simulink model "yoshi_rover_openloop"  (R2013b)
settings: Solver=ode3  SolverMode=SingleTasking  StartTime=0.0  StopTime=inf  RelTol=1e-3
model workspace (MAT data in the model file):
  rc = 0
  blc = -50
  brc = -50
  flc = 50
  frc = 20
undefined symbols (not defined in the file): DiscIntNeverNeededParam, sigbuilder_block, StatusID
libraries: arduinolib x5, simulink x5
settings Model: ExtModeTrigDuration=2  Creator=sbiagion  LastModifiedBy=scastro
settings DataIOCC: SignalLoggingSaveFormat=ModelDataLogs
settings OptimizationCC: OptimizeModelRefInitCode=on  LifeSpan=1
settings DebuggingCC: SolverPrmCheckMsg=none  MultiTaskDSMMsg=warning  MultiTaskCondExecSysMsg=none  StateNameClashWarn=warning
settings HardwareCC: ProdBitPerInt=16  ProdBitPerPointer=8  ProdIntDivRoundTo=Zero  ProdEndianess=LittleEndian  ProdWordSize=8  ProdHWDeviceType=Atmel->AVR
settings RTWCC: SystemTargetFile=realtime.tlc  GenerateMakefile=off  TemplateMakefile=realtime.tmf  Description=Run on Target Hardware  RTWVerbose=off  ProcessScript=realtime_make_rtw_hook  IncludeERTFirstTime=on
settings STFCustomTargetCC: TargetLibSuffix=.a  GenerateSampleERTMain=on  ERTCustomFileBanners=on  SupportNonInlinedSFcns=off  SupportVariableSizeSignals=on  MATLABClassNameForMDSCustomization=Simulink.SoftwareTarget.ERTCustomization  GRTInterface=off  SystemTargetFile=realtime.tlc
settings ERTTargetCC: CodeReplacementLibrary=ANSI_C  GenerateSampleERTMain=on  ParMdlRefBuildCompliant=off  CompOptLevelCompliant=off  ConcurrentExecutionCompliant=off  CombineOutputUpdateFcns=off  ERTFirstTimeCompliant=off  SupportContinuousTime=on  SupportVariableSizeSignals=on  ModelStepFunctionPrototypeControlCompliant=off  CPPClassGenCompliant=off  ExtModeTransport=3  ExtModeMexFile=ext_serial_win32_comm  ExtModeMexArgs=0 6 115200  InlinedParameterPlacement=NonHierarchical  ERTSrcFileBannerTemplate=realtime_code_template.cgt  ERTHdrFileBannerTemplate=realtime_code_template.cgt  ERTDataSrcFileTemplate=realtime_code_template.cgt  ERTDataHdrFileTemplate=realtime_code_template.cgt  ERTCustomFileTemplate=realtime_file_process.tlc

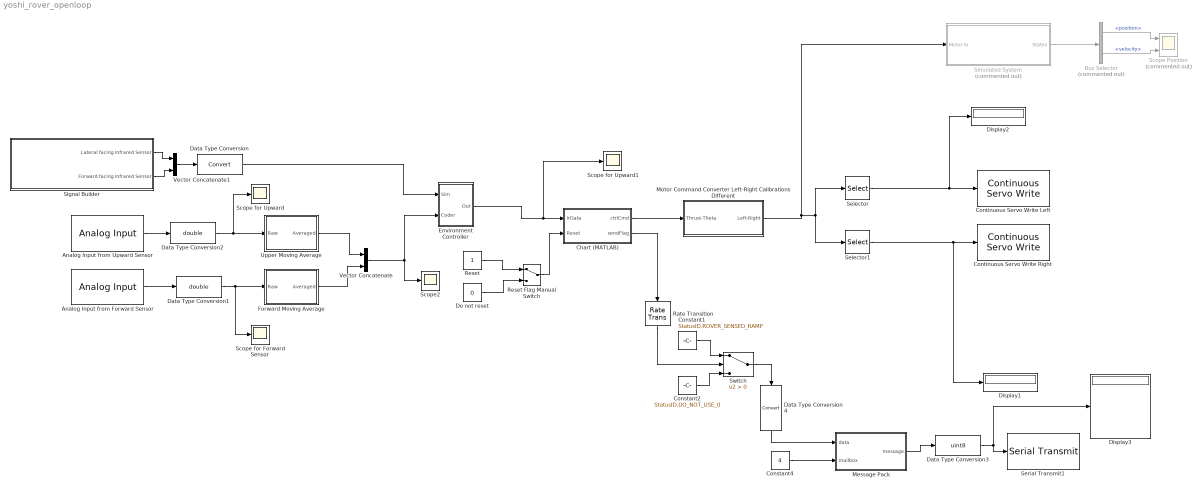
== system yoshi_rover_openloop ==
  Analog Input from Forward Sensor : arduinolib/Analog Input  pinNumber=1  sampleTime=0.01
  Analog Input from Upward Sensor : arduinolib/Analog Input  pinNumber=0  sampleTime=0.01
  Bus Selector : BusSelector  Commented=on  OutputSignals=position,velocity
  Chart (MATLAB) : Stateflow chart  TreatAsAtomicUnit=on
  Constant1 : Constant  Value=StatusID.ROVER_SENSED_RAMP  SampleTime=0.1
  Constant2 : Constant  Value=StatusID.DO_NOT_USE_0  SampleTime=0.1
  Constant4 : Constant  Value=4
  Continuous Servo Write Left : arduinolib/Continuous Servo Write  pinNumber=48
  Continuous Servo Write Right : arduinolib/Continuous Servo Write  pinNumber=49
  Data Type Conversion : DataTypeConversion
  Data Type Conversion1 : DataTypeConversion  OutDataTypeStr=double
  Data Type Conversion2 : DataTypeConversion  OutDataTypeStr=double
  Data Type Conversion3 : DataTypeConversion  OutDataTypeStr=uint8
  Data Type Conversion4 : DataTypeConversion
  Display1 : Display
  Display2 : Display
  Display3 : Display
  Do not reset : Constant  Value=0
  Environment Controller : Subsystem  mask(Environment Controller){}
      mask help: Simulink:masks:EnvironmentController_MD
      mask init:
      | switch_mode = rtwenvironmentmode(bdroot(gcbh)) || ...
      |     (exist('sldvisactive','file')~=0 && sldvisactive(bdroot(gcbh)));
  Forward Moving Average : Subsystem
  Message Pack : Subsystem
  Motor Command Converter Left-Right Calibrations Different : Subsystem  AncestorBlock="battlebots_library/Motor Control/Motor Command Converter  Left-Right Calibrations Different"  mask{fcl=flc, fcr=frc, rc=rc, bcl=blc, bcr=brc}
      mask prompts: fcl "Forward Left"; fcr "Forward Right"; rc "Rest"; bcl "Backward Left"; bcr "Backward Right"
  Rate Transition : RateTransition  OutPortSampleTime=0.1
  Reset : Constant
  Reset Flag Manual Switch : ManualSwitch
  Scope Position : Scope  Commented=on  NumInputPorts=2
      settings: ShowLegends=on  YMin=-5~-0.5  YMax=5~1  SaveName=ScopeData3
  Scope for Forward Sensor : Scope
      settings: YMin=0  YMax=1000
  Scope for Upward : Scope
      settings: YMin=25  YMax=525  SaveName=ScopeData6
  Scope for Upward1 : Scope
      settings: ShowLegends=on  YMin=0  YMax=700  SaveName=RoverSensorData
  Scope2 : Scope
      settings: ShowLegends=on  YMin=25  YMax=600  SaveName=ScopeData2
  Selector : Selector  InputPortWidth=2  IndexOptions=Index vector (dialog)  Indices=1  OutputSizes=1
  Selector1 : Selector  InputPortWidth=2  IndexOptions=Index vector (dialog)  Indices=2  OutputSizes=1
  Serial Transmit1 : arduinolib/Serial Transmit  portNumber=1
  Signal Builder : Subsystem  Tag=STV Subsys  LoadFcn=sigbuilder_block('load');  StartFcn=sigbuilder_block('start');  StopFcn=sigbuilder_block('stop');  ClipboardFcn=sigbuilder_block('clipboard');  mask(Sigbuilder block){}
      mask help: Simulink:masks:SigbuilderBlock_MD
      mask init:
      | if ~strcmp(get_param(bdroot(gcbh),'SimulationStatus'),'stopped') tuvar = sigbuilder_block('maskInit'); end
      settings: CopyFcn=sigbuilder_block('copy');  DeleteFcn=sigbuilder_block('delete');  ModelCloseFcn=sigbuilder_block('modelClose');  PreSaveFcn=sigbuilder_block('preSave');  PauseFcn=sigbuilder_block('pause');  ContinueFcn=sigbuilder_block('continue');  NameChangeFcn=sigbuilder_block('namechange');  OpenFcn=sigbuilder_block('open',[36 193.034 550.552 399.724 ]);  CloseFcn=sigbuilder_block('close');
      mask Display: plot(0, 0, 100, 100,[2, 2, 32, 32, 2], [68, 8, 8, 68, 68],[32, 2], [38, 38], [32, 19, 2],[53, 60, 44], [32, 17, 17, 2],[16, 16, 31, 31]);txt = getActiveGroup(gcbh);text(2, 100, txt,'verticalAlignment', 'top');
  Simulated System : Subsystem  Commented=on  AncestorBlock=battlebots_library/Simulation/Simulated System1  mask{max2vel=1, xm_initial_ft=0, ym_initial_ft=0, om_initial_rad=0, wheelbase_ft=1}
      mask prompts: max2vel "Gain to convert maximum command to velocity"; xm_initial_ft "Initial x position in ft"; ym_initial_ft "Initial y position in ft"; om_initial_rad "Initial orientation in radians"; wheelbase_ft "Wheelbase in ft"
  Switch : Switch  Criteria=u2 > Threshold
  Upper Moving Average : Subsystem
  Vector Concatenate : Concatenate
  Vector Concatenate1 : Concatenate
  wires:
  Analog Input from Upward Sensor/1 -> Data Type Conversion2/1
  Environment Controller/1(Out) -> Scope for Upward1/1, Chart (MATLAB)/1(irData)
  Data Type Conversion/1 -> Environment Controller/1(Sim)
  Signal Builder/2(Forward facing Infrared Sensor) -> Vector Concatenate1/2
  Signal Builder/1(Lateral facing Infrared Sensor) -> Vector Concatenate1/1
  Vector Concatenate1/1 -> Data Type Conversion/1
  Motor Command Converter Left-Right Calibrations Different/1(Left-Right) -> Simulated System/1(Motor In), Selector1/1, Selector/1
  Vector Concatenate/1 -> Scope2/1, Environment Controller/2(Coder)
  Analog Input from Forward Sensor/1 -> Data Type Conversion1/1
  Data Type Conversion2/1 -> Scope for Upward/1, Upper Moving Average/1(Raw)
  Selector1/1 -> Display1/1, Continuous Servo Write Right/1
  Selector/1 -> Continuous Servo Write Left/1, Display2/1
  Simulated System/1(States) -> Bus Selector/1
  Bus Selector/1 -> Scope Position/1  "<position>"
  Bus Selector/2 -> Scope Position/2  "<velocity>"
  Chart (MATLAB)/1(ctrlCmd) -> Motor Command Converter Left-Right Calibrations Different/1(Thrust-Theta)
  Data Type Conversion1/1 -> Scope for Forward Sensor/1, Forward Moving Average/1(Raw)
  Forward Moving Average/1("Averaged ") -> Vector Concatenate/2
  Upper Moving Average/1(Averaged) -> Vector Concatenate/1
  Reset Flag Manual Switch/1 -> Chart (MATLAB)/2(Reset)
  Reset/1 -> Reset Flag Manual Switch/1
  Do not reset/1 -> Reset Flag Manual Switch/2
  Constant4/1 -> Message Pack/2(mailbox)
  Message Pack/1(message) -> Data Type Conversion3/1
  Data Type Conversion3/1 -> Serial Transmit1/1, Display3/1
  Chart (MATLAB)/2(sendFlag) -> Rate Transition/1
  Constant1/1 -> Switch/1
  Constant2/1 -> Switch/3
  Switch/1 -> Data Type Conversion4/1
  Data Type Conversion4/1 -> Message Pack/1(data)
  Rate Transition/1 -> Switch/2

== system yoshi_rover_openloop/Environment Controller ==
  Sim : Inport
  Coder : Inport  Port=2
  Environment Switch : Switch  DisableCoverage=on  Criteria=u2 ~= 0  ZeroCross=off  InputSameDT=on
  Numerical Unity : SignalConversion
  Switch Control : Constant  DisableCoverage=on  Value=switch_mode  OutDataTypeStr=boolean
  Out : Outport
  wires:
  Numerical Unity/1 -> Out/1
  Coder/1 -> Environment Switch/3
  Environment Switch/1 -> Numerical Unity/1
  Switch Control/1 -> Environment Switch/2
  Sim/1 -> Environment Switch/1

== system yoshi_rover_openloop/Forward Moving Average ==
  Raw : Inport
  Gain : Gain  Gain=1/15
  Sum of Elements : Sum  Inputs=+
  Tapped Delay : simulink/Discrete/Tapped Delay  vinit=0.0  samptime=-1  NumDelays=15  DelayOrder=Oldest  includeCurrent=off
  "Averaged " : Outport
  wires:
  Sum of Elements/1 -> Gain/1
  Tapped Delay/1 -> Sum of Elements/1
  Gain/1 -> "Averaged "/1
  Raw/1 -> Tapped Delay/1

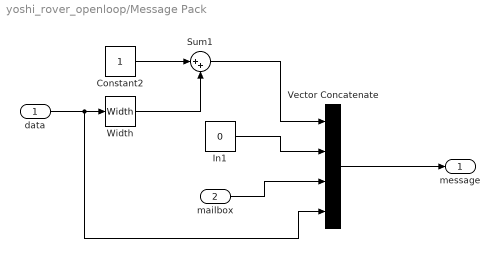
== system yoshi_rover_openloop/Message Pack ==
  data : Inport
  mailbox : Inport  Port=2
  Constant2 : Constant
  In1 : Constant  Value=0
  Sum1 : Sum  Inputs=|++
  Vector Concatenate : Concatenate  NumInputs=4
  Width : Width
  message : Outport
  wires:
  Constant2/1 -> Sum1/1
  In1/1 -> Vector Concatenate/2
  data/1 -> Vector Concatenate/4, Width/1
  Vector Concatenate/1 -> message/1
  mailbox/1 -> Vector Concatenate/3
  Sum1/1 -> Vector Concatenate/1
  Width/1 -> Sum1/2

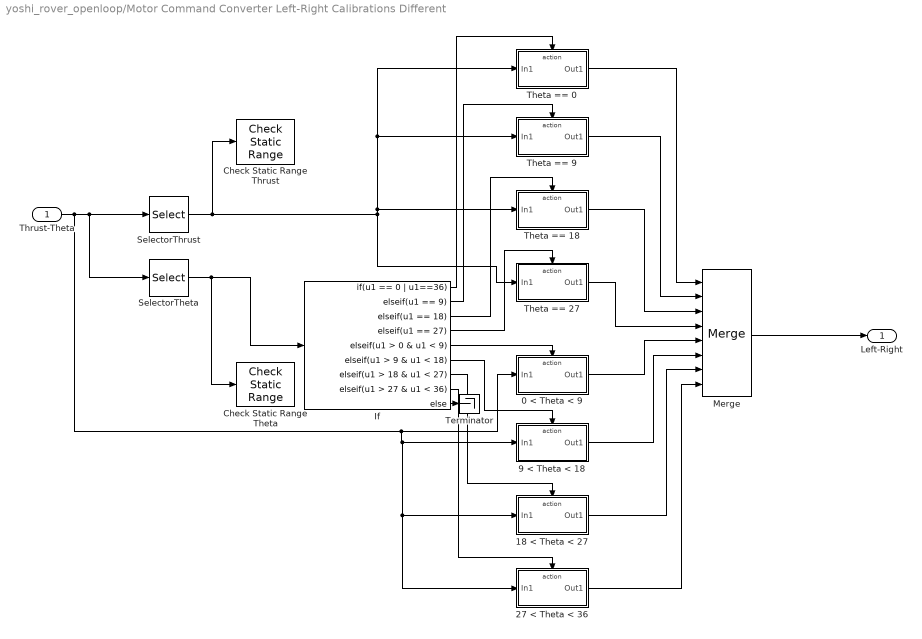
== system yoshi_rover_openloop/Motor Command Converter Left-Right Calibrations Different ==
  Thrust-Theta : Inport
  0 < Theta < 9 : Subsystem  TreatAsAtomicUnit=on
  18 < Theta < 27 : Subsystem  TreatAsAtomicUnit=on
  27 < Theta < 36 : Subsystem  TreatAsAtomicUnit=on
  9 < Theta < 18 : Subsystem  TreatAsAtomicUnit=on
  Check Static Range Theta : simulink/Model Verification/Check  Static Range  Description=0 <= u <= 36  max=36  max_included=on  min=0  min_included=on  enabled=on  callback=error('Theta Out of Range. Must be between 0 and 36, inclusively.')  stopWhenAssertionFail=on  export=off  icon=graphic
  Check Static Range Thrust : simulink/Model Verification/Check  Static Range  Description=0 <= u <= 9  max=9  max_included=on  min=0  min_included=on  enabled=on  callback=error('Thrust Out of Range. Must be between 0 and 9, inclusively.')  stopWhenAssertionFail=on  export=off  icon=graphic
  If : If  IfExpression=u1 == 0 | u1==36  ElseIfExpressions=u1 == 9, u1 == 18, u1 == 27, u1 > 0 & u1 < 9, u1 > 9 & u1 < 18, u1 > 18 & u1 < 27, u1 > 27 & u1 < 36
  Merge : Merge  Inputs=8
  "SelectorTheta " : Selector  InputPortWidth=2  IndexOptions=Index vector (dialog)  Indices=[2]  OutputSizes=1
  SelectorThrust : Selector  InputPortWidth=2  IndexOptions=Index vector (dialog)  Indices=[1]  OutputSizes=1
  Terminator : Terminator
  Theta == 0 : Subsystem  TreatAsAtomicUnit=on
  Theta == 18 : Subsystem  TreatAsAtomicUnit=on
  Theta == 27 : Subsystem  TreatAsAtomicUnit=on
  Theta == 9 : Subsystem  TreatAsAtomicUnit=on
  Left-Right : Outport
  wires:
  If/9 -> Terminator/1
  Thrust-Theta/1 -> 27 < Theta < 36/1(In1), 18 < Theta < 27/1(In1), 9 < Theta < 18/1(In1), 0 < Theta < 9/1(In1), "SelectorTheta "/1, SelectorThrust/1
  "SelectorTheta "/1 -> If/1, Check Static Range Theta/1
  If/1 -> Theta == 0/Action
  If/2 -> Theta == 9/Action
  If/3 -> Theta == 18/Action
  If/4 -> Theta == 27/Action
  If/5 -> 0 < Theta < 9/Action
  If/6 -> 9 < Theta < 18/Action
  If/7 -> 18 < Theta < 27/Action
  If/8 -> 27 < Theta < 36/Action
  SelectorThrust/1 -> Theta == 0/1(In1), Theta == 9/1(In1), Theta == 18/1(In1), Theta == 27/1(In1), Check Static Range Thrust/1
  Theta == 0/1(Out1) -> Merge/1
  Theta == 9/1(Out1) -> Merge/2
  Theta == 18/1(Out1) -> Merge/3
  Merge/1 -> Left-Right/1
  Theta == 27/1(Out1) -> Merge/4
  0 < Theta < 9/1(Out1) -> Merge/5
  9 < Theta < 18/1(Out1) -> Merge/6
  18 < Theta < 27/1(Out1) -> Merge/7
  27 < Theta < 36/1(Out1) -> Merge/8

== system yoshi_rover_openloop/Signal Builder ==
  Demux : Demux  Tag=STV Demux  Outputs=2
  FromWs : FromWorkspace  Tag=STV FromWs  VariableName=tuvar  OutputAfterFinalValue=Holding final value
      SigBuilderData=|
      | common.afterFinalStr = 'Hold final value'
      | common.sampleTime = '-1'
      | dataSet.timeRange = [0 20]
      | dataSet.name = 'Group 1'
      | sbobj.Groups.Name = 'Group 1'
      | sbobj.Groups.Signals(1).Name = 'Lateral facing Infrared Sensor'
      | sbobj.Groups.Signals(1).XData = [0 5 5 7 7 20]
      | sbobj.Groups.Signals(1).YData = [200 199.5 402 400 200 200]
      | sbobj.Groups.Signals(2).Name = 'Forward facing Infrared Sensor'
      | sbobj.Groups.Signals(2).XData = [0 12 16 20]
      | sbobj.Groups.Signals(2).YData = [200 200 450 496]
      | sbobj.Groups.TimeRange = [0 20]
  Lateral facing Infrared Sensor : Outport  Tag=STV Outport
  Forward facing Infrared Sensor : Outport  Tag=STV Outport  Port=2
  wires:
  Demux/1 -> Lateral facing Infrared Sensor/1
  FromWs/1 -> Demux/1
  Demux/2 -> Forward facing Infrared Sensor/1

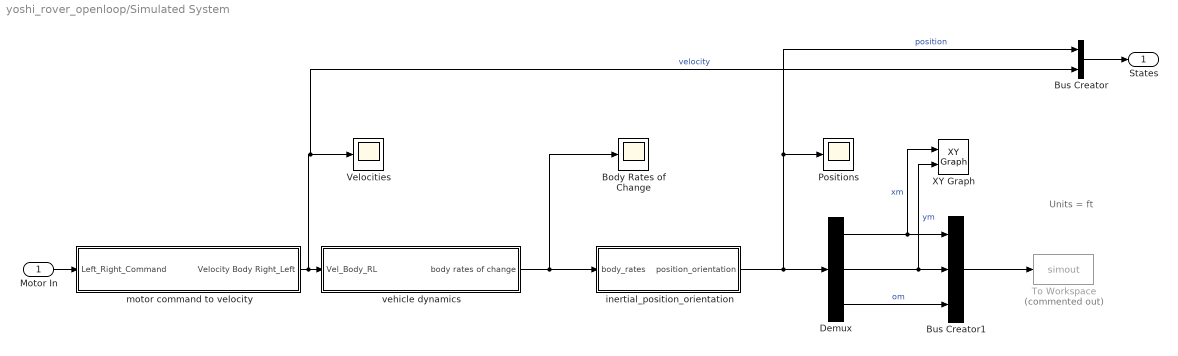
== system yoshi_rover_openloop/Simulated System ==
  note: Units = ft
  Motor In : Inport
  Body Rates of Change : Scope
      settings: ShowLegends=on  SaveName=ScopeData5
  Bus Creator : BusCreator  Inputs=2
  Bus Creator1 : BusCreator  Inputs=3
  Demux : Demux  Outputs=3
  Positions : Scope
      settings: ShowLegends=on  SaveName=ScopeData3
  To Workspace : ToWorkspace  Commented=on  VariableName=simout  SampleTime=-1  SaveFormat=Timeseries
  Velocities : Scope
      settings: ShowLegends=on  YMin=-1  YMax=1  SaveName=ScopeData4
  XY Graph : simulink/Sinks/XY Graph  xmin=-2  xmax=5  ymin=-5  ymax=5  st=1
  inertial_position_orientation : Subsystem
  motor command to velocity : Subsystem
  vehicle dynamics : Subsystem
  States : Outport
  wires:
  Bus Creator/1 -> States/1
  vehicle dynamics/1(body rates of change) -> Body Rates of Change/1, inertial_position_orientation/1(body_rates)
  inertial_position_orientation/1(position_orientation) -> Positions/1, Bus Creator/1, Demux/1  "position"
  motor command to velocity/1(Velocity Body Right_Left) -> Velocities/1, Bus Creator/2, vehicle dynamics/1(Vel_Body_RL)  "velocity"
  Motor In/1 -> motor command to velocity/1(Left_Right_Command)
  Demux/3 -> Bus Creator1/3  "om"
  Demux/2 -> Bus Creator1/2, XY Graph/2  "ym"
  Demux/1 -> Bus Creator1/1, XY Graph/1  "xm"
  Bus Creator1/1 -> To Workspace/1

== system yoshi_rover_openloop/Upper Moving Average ==
  Raw : Inport
  Gain : Gain  Gain=1/5
  Sum of Elements : Sum  Inputs=+
  Tapped Delay : simulink/Discrete/Tapped Delay  vinit=0.0  samptime=-1  NumDelays=5  DelayOrder=Oldest  includeCurrent=off
  Averaged : Outport
  wires:
  Raw/1 -> Tapped Delay/1
  Gain/1 -> Averaged/1
  Tapped Delay/1 -> Sum of Elements/1
  Sum of Elements/1 -> Gain/1

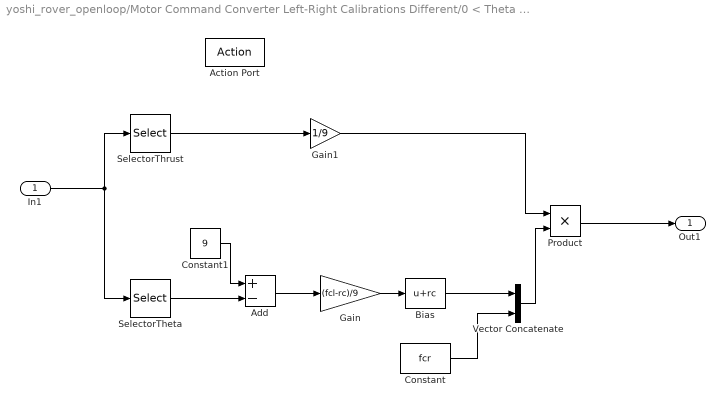
== system yoshi_rover_openloop/Motor Command Converter Left-Right Calibrations Different/0 < Theta < 9 ==
  In1 : Inport
  Action Port : ActionPort  ActionType=elseif
  Add : Sum  Inputs=+-
  Bias : Bias  Bias=rc
  Constant : Constant  Value=fcr  OutDataTypeStr=Inherit: Inherit via back propagation
  Constant1 : Constant  Value=9
  Gain : Gain  Gain=(fcl-rc)/9  OutDataTypeStr=Inherit: Same as input
  Gain1 : Gain  Gain=1/9  OutDataTypeStr=Inherit: Same as input
  Product : Product  OutDataTypeStr=Inherit: Same as first input
  SelectorTheta : Selector  InputPortWidth=2  IndexOptions=Index vector (dialog)  Indices=2  OutputSizes=1
  SelectorThrust : Selector  InputPortWidth=2  IndexOptions=Index vector (dialog)  Indices=1  OutputSizes=1
  Vector Concatenate : Concatenate
  Out1 : Outport
  wires:
  Add/1 -> Gain/1
  Constant1/1 -> Add/1
  SelectorTheta/1 -> Add/2
  Constant/1 -> Vector Concatenate/2
  In1/1 -> SelectorTheta/1, SelectorThrust/1
  SelectorThrust/1 -> Gain1/1
  Gain1/1 -> Product/1
  Vector Concatenate/1 -> Product/2
  Bias/1 -> Vector Concatenate/1
  Gain/1 -> Bias/1
  Product/1 -> Out1/1

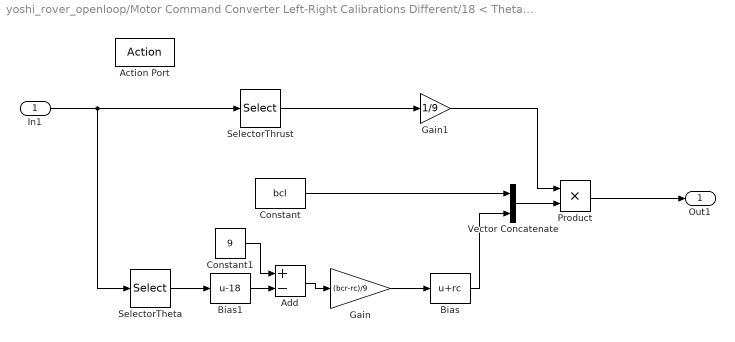
== system yoshi_rover_openloop/Motor Command Converter Left-Right Calibrations Different/18 < Theta < 27 ==
  In1 : Inport
  Action Port : ActionPort  ActionType=elseif
  Add : Sum  Inputs=+-
  Bias : Bias  Bias=rc
  Bias1 : Bias  Bias=-18
  Constant : Constant  Value=bcl  OutDataTypeStr=Inherit: Inherit via back propagation
  Constant1 : Constant  Value=9
  Gain : Gain  Gain=(bcr-rc)/9  OutDataTypeStr=Inherit: Same as input
  Gain1 : Gain  Gain=1/9  OutDataTypeStr=Inherit: Same as input
  Product : Product  OutDataTypeStr=Inherit: Same as first input
  SelectorTheta : Selector  InputPortWidth=2  IndexOptions=Index vector (dialog)  Indices=2  OutputSizes=1
  SelectorThrust : Selector  InputPortWidth=2  IndexOptions=Index vector (dialog)  Indices=1  OutputSizes=1
  Vector Concatenate : Concatenate
  Out1 : Outport
  wires:
  Constant1/1 -> Add/1
  Add/1 -> Gain/1
  Bias1/1 -> Add/2
  In1/1 -> SelectorTheta/1, SelectorThrust/1
  Gain/1 -> Bias/1
  SelectorTheta/1 -> Bias1/1
  SelectorThrust/1 -> Gain1/1
  Product/1 -> Out1/1
  Gain1/1 -> Product/1
  Vector Concatenate/1 -> Product/2
  Constant/1 -> Vector Concatenate/1
  Bias/1 -> Vector Concatenate/2

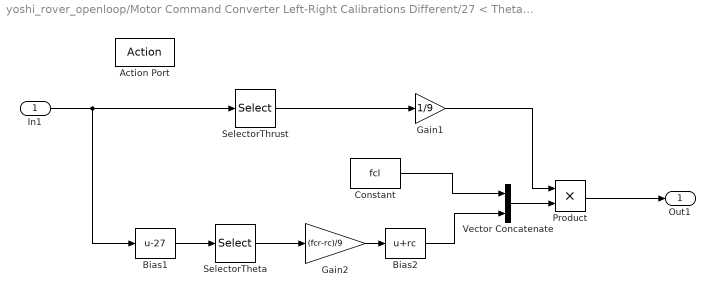
== system yoshi_rover_openloop/Motor Command Converter Left-Right Calibrations Different/27 < Theta < 36 ==
  In1 : Inport
  Action Port : ActionPort  ActionType=elseif
  Bias1 : Bias  Bias=-27
  Bias2 : Bias  Bias=rc
  Constant : Constant  Value=fcl  OutDataTypeStr=Inherit: Inherit via back propagation
  Gain1 : Gain  Gain=1/9  OutDataTypeStr=Inherit: Same as input
  Gain2 : Gain  Gain=(fcr-rc)/9  OutDataTypeStr=Inherit: Same as input
  Product : Product  OutDataTypeStr=Inherit: Same as first input
  SelectorTheta : Selector  InputPortWidth=2  IndexOptions=Index vector (dialog)  Indices=2  OutputSizes=1
  SelectorThrust : Selector  InputPortWidth=2  IndexOptions=Index vector (dialog)  Indices=1  OutputSizes=1
  Vector Concatenate : Concatenate
  Out1 : Outport
  wires:
  In1/1 -> Bias1/1, SelectorThrust/1
  Constant/1 -> Vector Concatenate/1
  SelectorThrust/1 -> Gain1/1
  Product/1 -> Out1/1
  Gain1/1 -> Product/1
  Vector Concatenate/1 -> Product/2
  Bias1/1 -> SelectorTheta/1
  SelectorTheta/1 -> Gain2/1
  Gain2/1 -> Bias2/1
  Bias2/1 -> Vector Concatenate/2

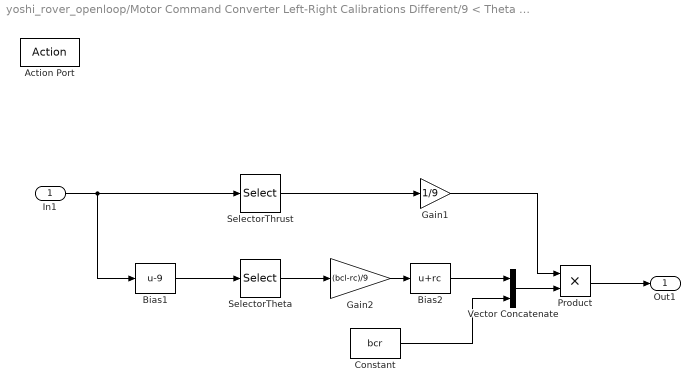
== system yoshi_rover_openloop/Motor Command Converter Left-Right Calibrations Different/9 < Theta < 18 ==
  In1 : Inport
  Action Port : ActionPort  ActionType=elseif
  Bias1 : Bias  Bias=-9
  Bias2 : Bias  Bias=rc
  Constant : Constant  Value=bcr  OutDataTypeStr=Inherit: Inherit via back propagation
  Gain1 : Gain  Gain=1/9  OutDataTypeStr=Inherit: Same as input
  Gain2 : Gain  Gain=(bcl-rc)/9  OutDataTypeStr=Inherit: Same as input
  Product : Product  OutDataTypeStr=Inherit: Same as first input
  SelectorTheta : Selector  InputPortWidth=2  IndexOptions=Index vector (dialog)  Indices=2  OutputSizes=1
  SelectorThrust : Selector  InputPortWidth=2  IndexOptions=Index vector (dialog)  Indices=1  OutputSizes=1
  Vector Concatenate : Concatenate
  Out1 : Outport
  wires:
  Constant/1 -> Vector Concatenate/2
  In1/1 -> Bias1/1, SelectorThrust/1
  Bias1/1 -> SelectorTheta/1
  Bias2/1 -> Vector Concatenate/1
  SelectorThrust/1 -> Gain1/1
  Product/1 -> Out1/1
  Gain1/1 -> Product/1
  Vector Concatenate/1 -> Product/2
  SelectorTheta/1 -> Gain2/1
  Gain2/1 -> Bias2/1

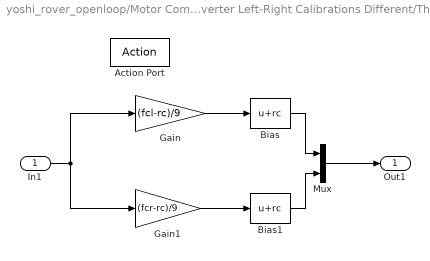
== system yoshi_rover_openloop/Motor Command Converter Left-Right Calibrations Different/Theta == 0 ==
  In1 : Inport
  Action Port : ActionPort  ActionType=then
  Bias : Bias  Bias=rc
  Bias1 : Bias  Bias=rc
  Gain : Gain  Gain=(fcl-rc)/9  OutDataTypeStr=Inherit: Inherit via back propagation
  Gain1 : Gain  Gain=(fcr-rc)/9  OutDataTypeStr=Inherit: Inherit via back propagation
  Mux : Mux  Inputs=2
  Out1 : Outport
  wires:
  Bias/1 -> Mux/1
  In1/1 -> Gain/1, Gain1/1
  Gain/1 -> Bias/1
  Gain1/1 -> Bias1/1
  Bias1/1 -> Mux/2
  Mux/1 -> Out1/1

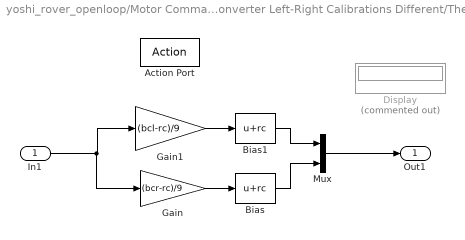
== system yoshi_rover_openloop/Motor Command Converter Left-Right Calibrations Different/Theta == 18 ==
  In1 : Inport
  Action Port : ActionPort  ActionType=elseif
  Bias : Bias  Bias=rc
  Bias1 : Bias  Bias=rc
  Display : Display  Commented=on
  Gain : Gain  Gain=(bcr-rc)/9  OutDataTypeStr=Inherit: Inherit via back propagation
  Gain1 : Gain  Gain=(bcl-rc)/9  OutDataTypeStr=Inherit: Inherit via back propagation
  Mux : Mux  Inputs=2
  Out1 : Outport
  wires:
  Mux/1 -> Out1/1
  Gain1/1 -> Bias1/1
  Bias1/1 -> Mux/1
  In1/1 -> Gain/1, Gain1/1
  Gain/1 -> Bias/1
  Bias/1 -> Mux/2

== system yoshi_rover_openloop/Motor Command Converter Left-Right Calibrations Different/Theta == 27 ==
  In1 : Inport
  Action Port : ActionPort  ActionType=elseif
  Bias : Bias  Bias=rc
  Bias1 : Bias  Bias=rc
  Gain : Gain  Gain=(fcl-rc)/9  OutDataTypeStr=Inherit: Same as input
  Gain1 : Gain  Gain=(bcr-rc)/9  OutDataTypeStr=Inherit: Same as input
  Mux : Mux  Inputs=2
  Out1 : Outport
  wires:
  Bias/1 -> Mux/1
  In1/1 -> Gain/1, Gain1/1
  Gain/1 -> Bias/1
  Gain1/1 -> Bias1/1
  Bias1/1 -> Mux/2
  Mux/1 -> Out1/1

== system yoshi_rover_openloop/Motor Command Converter Left-Right Calibrations Different/Theta == 9 ==
  In1 : Inport
  Action Port : ActionPort  ActionType=elseif
  Bias : Bias  Bias=rc
  Bias1 : Bias  Bias=rc
  Gain : Gain  Gain=(bcl-rc)/9  OutDataTypeStr=Inherit: Inherit via back propagation
  Gain1 : Gain  Gain=(fcr-rc)/9  OutDataTypeStr=Inherit: Inherit via back propagation
  Mux : Mux  Inputs=2
  Out1 : Outport
  wires:
  Bias/1 -> Mux/1
  In1/1 -> Gain/1, Gain1/1
  Gain/1 -> Bias/1
  Gain1/1 -> Bias1/1
  Bias1/1 -> Mux/2
  Mux/1 -> Out1/1

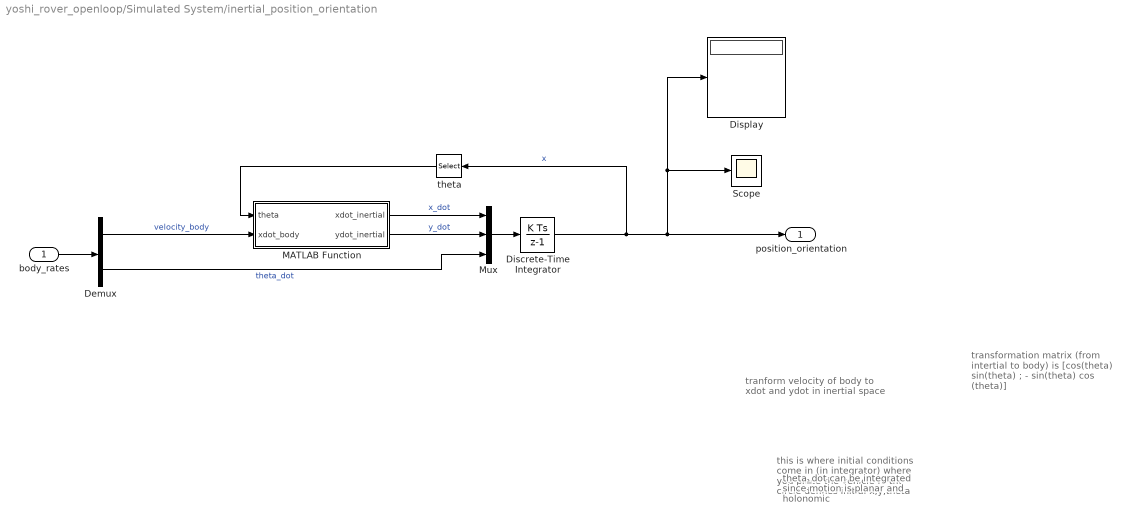
== system yoshi_rover_openloop/Simulated System/inertial_position_orientation ==
  note: transformation matrix (from intertial to body) is [cos(theta) sin(theta) ; - sin(theta) cos (theta)]
  note: tranform velocity of body to xdot and ydot in inertial space
  note: this is where initial conditions come in (in integrator)
      | where you place the vehicle in the circle defines initial x,y,theta
  note: theta_dot can be integrated since motion is planar and holonomic
  body_rates : Inport
  Demux : Demux  Outputs=2
  Discrete-Time Integrator : DiscreteIntegrator  InitialCondition=[xm_initial_ft ym_initial_ft om_initial_rad]  SampleTime=-1  ICPrevOutput=DiscIntNeverNeededParam  ICPrevScaledInput=DiscIntNeverNeededParam
  Display : Display
  MATLAB Function : MATLAB Function  TreatAsAtomicUnit=on
  Mux : Mux  Inputs=3
  Scope : Scope
      settings: ShowLegends=on  YMin=-2  YMax=32  SaveName=ScopeData2
  theta : Selector  InputPortWidth=3  IndexOptions=Index vector (dialog)  Indices=[3]  OutputSizes=1
  position_orientation : Outport
  wires:
  MATLAB Function/1(xdot_inertial) -> Mux/1  "x_dot"
  MATLAB Function/2(ydot_inertial) -> Mux/2  "y_dot"
  Demux/2 -> Mux/3  "theta_dot"
  Demux/1 -> MATLAB Function/2(xdot_body)  "velocity_body"
  theta/1 -> MATLAB Function/1(theta)
  Mux/1 -> Discrete-Time Integrator/1
  Discrete-Time Integrator/1 -> position_orientation/1, Display/1, Scope/1, theta/1  "x"
  body_rates/1 -> Demux/1

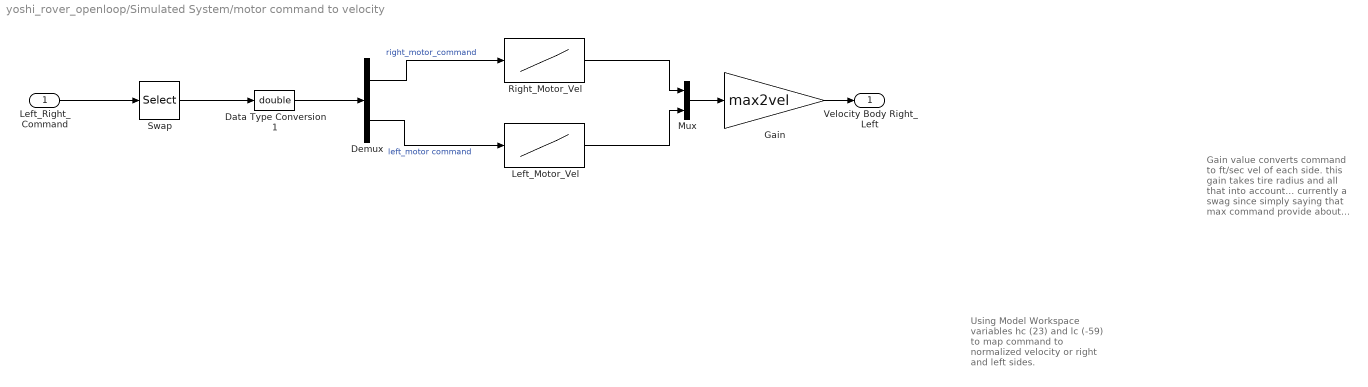
== system yoshi_rover_openloop/Simulated System/motor command to velocity ==
  note: Using Model Workspace variables hc (23) and lc (-59)
      | to map command to normalized velocity or right and left sides.
  note: Gain value converts command to ft/sec vel
      | of each side.  this gain takes tire radius and all that
      | into account... currently a swag since simply saying that max
      | command provide about 1 ft/sec velocity.
  Left_Right_Command : Inport
  Data Type Conversion1 : DataTypeConversion  OutDataTypeStr=double
  Demux : Demux  Outputs=2
  Gain : Gain  Gain=max2vel  ParamDataTypeStr=single  OutDataTypeStr=double
  Left_Motor_Vel : Lookup_n-D  NumberOfTableDimensions=1  BreakpointsForDimension1=[blc rc flc]  Table=[-1 0 1]  RndMeth=Simplest  InputSameDT=on
  Mux : Mux  Inputs=2
  Right_Motor_Vel : Lookup_n-D  NumberOfTableDimensions=1  BreakpointsForDimension1=[brc rc frc]  Table=[-1 0 1]  RndMeth=Simplest  InputSameDT=on
  Swap : Selector  InputPortWidth=2  IndexOptions=Index vector (dialog)  Indices=[2 1]  OutputSizes=1
  Velocity Body Right_Left : Outport  OutDataTypeStr=double
  wires:
  Data Type Conversion1/1 -> Demux/1
  Swap/1 -> Data Type Conversion1/1
  Demux/2 -> Left_Motor_Vel/1  "left_motor command"
  Demux/1 -> Right_Motor_Vel/1  "right_motor_command"
  Left_Right_Command/1 -> Swap/1
  Mux/1 -> Gain/1
  Right_Motor_Vel/1 -> Mux/1
  Left_Motor_Vel/1 -> Mux/2
  Gain/1 -> Velocity Body Right_Left/1

== system yoshi_rover_openloop/Simulated System/vehicle dynamics ==
  note: [vcm thetadot]
  note: velocity of the vehicle (ft/s) (point mass in the middle) in the body coord
      | system is the sum of velocities on each side divided by 2
  note: theta_dot (rad/s) is equal to the difference (right minus left)
      | divided by the wheel base.  Positive values are a
      | positive theta dot (z axis pointing to ceiling from floor)
  Vel_Body_RL : Inport
  Demux : Demux  Outputs=2
  Gain : Gain  Gain=1/2
  Gain1 : Gain  Gain=1/wheelbase_ft
  Mux : Mux  Inputs=2
  Sum of Elements : Sum  Inputs=+
  Sum of Elements1 : Sum  Inputs=+-
  body rates of change : Outport
  wires:
  Gain1/1 -> Mux/2
  Sum of Elements1/1 -> Gain1/1
  Demux/2 -> Sum of Elements1/2
  Demux/1 -> Sum of Elements1/1
  Gain/1 -> Mux/1
  Mux/1 -> body rates of change/1
  Sum of Elements/1 -> Gain/1
  Vel_Body_RL/1 -> Sum of Elements/1, Demux/1

== matlab function yoshi_rover_openloop/Simulated System/inertial_position_orientation/MATLAB Function ==
  data: theta input; xdot_inertial output; xdot_body input; ydot_inertial output
function [xdot_inertial, ydot_inertial]  = fcn(theta, xdot_body)
%#codegen

% transformation from intertial to body
T_bi = [cos(theta) sin(theta);
        -sin(theta) cos(theta)];
    
% note transpose of T since moving from body to inertial
vel_i = T_bi'*[xdot_body;0];

xdot_inertial = vel_i(1);
ydot_inertial = vel_i(2);

== stateflow chart yoshi_rover_openloop/Chart (MATLAB) ==
  note: 1.5 0
  note: 470
  state waitForMario
    en, du:
    sendFlag=0;
    ctrlCmd=[0 0];
  state MoveForward
    entry:
    ctrlCmd=[3.5 0];
  state Stop
    entry:
    ctrlCmd=[0 0];
    sendFlag=1;
  (default) -> waitForMario
  MoveForward -> Stop : [irData(2)>430]
  waitForMario -> MoveForward : [irData(1)>200]
  Stop -> waitForMario : [Reset == 1]
  data: irData input; ctrlCmd output double size=[1 2]; Reset input size=1; sendFlag output
